simulink model "BEVplantModel"  (R2022b)
settings: Solver=daessc  StartTime=0  StopTime=50  RelTol=1e-3
PreLoadFcn:
  | % Load all parameters
  | BEVplantModelParam;
undefined symbols (not defined in the file): battery, cabin_T_init, coolant_pipe_D, coolant_valve_D_ratio_max, coolant_valve_D_ratio_min, coolant_valve_displacement, electricDrive, max_torque, vehicle, vehicleThermal
libraries: fl_lib x292, nesl_utility x67, SimscapeFluids_lib x15, ee_lib x11, sdl_lib x8, BatteryCurrentManagement x3, slpidlib x3, simulink x2, BatteryThermalManagement x1, autolibshared x1
(part 5 of 10)

== system BEVplantModel/Vehicle/Rear Motor (EM2) ==
  s : Inport
  Bus Creator : BusCreator  Inputs=2
  Bus Selector : BusSelector  OutputSignals=EM2Trq,Batt
  Bus Selector1 : BusSelector  OutputSignals=EM1rpm
  Coolant Jacket : SimscapeFluids_lib/Thermal Liquid/Pipes & Fittings/Pipe (TL)  dynamic_compressibility=1  inertia=0  num_segments=1  pipe_length=0.4 m  area=4 * pi * vehicleThermal.coolant_channel_D^2 / 4 m^2  wall_spec=1  Dh=vehicleThermal.coolant_channel_D m  wall_compliance=1.2e-6 m/MPa  wall_time_constant=0.01 s  elevation_spec=foundation.enum.constant_variable.constant  elevation_gain=0 m  g=9.81 m/s^2  pressure_loss_spec=1  local_pressure_loss_spec=fluids.thermal_liquid.pipes_fittings.enum.LocalLossSpec.AggregateLength  length_add=20 * vehicleThermal.coolant_channel_D * 4 m  loss_coefficient=0.1  roughness=1.5e-5 m  Re_friction_TLU=[ 400 1000 1.5e+3 3e+3 4e+3 6e+3 1e+4 2e+4 4e+4 6e+4 1e+5 1e+8 ]  friction_factor_TLU=[ 0.264 0.112 0.07099999999999999 0.0417 0.0387 0.0268 0.025 0.0232 0.0226 0.022 0.0214 0.0214 ]  shape_factor=64  Re_lam=100  Re_tur=500  mdot_nominal=[ 0.1 1 ] kg/s  p_diff_nominal=[ 0.001 0.01 ] MPa  mdot_threshold=1e-6 kg/s  heat_transfer_spec=4  mdot_nominal_heat=[ 0.1 1 ] kg/s  T_in_nominal=[ 293.15 293.15 ] K  T_out_nominal=[ 300 300 ] K  p_in_nominal_heat=[ 0.101325 0.101325 ] MPa  T_wall_nominal=[ 303.15 303.15 ] K  a_coeff=0.3  b_Re_power=0.8  c_Pr_power=0.33  Nu_lam=3.66  Re_Colburn_TLU=[ 100 150 1000 ]  Colburn_factor_TLU=[ 0.019 0.013 0.002 ]  Re_Nu_TLU=[ 100 150 1000 ]  Pr_Nu_TLU=[ 1 10 ]  Nu_TLU=[ 3.72 4.21; 3.75 4.44; 4.21 7.15 ]  T0_vec=vehicleThermal.coolant_T_init K  p0_vec=vehicleThermal.coolant_p_init MPa  mdot0=0.1 kg/s
  Emotor : Subsystem
      settings: PortSchema="{\"entries\":[{\"content\":{\"sides\":[{\"content\":{\"connectorIds\":[\"LConn1\",\"In1\"]},\"type\":\"ConnectorPlacement.EquallySpacedRectSide\",\"uuid\":\"4c01f4e7-db0d-4a8e-9bf8-0007797f2983\"},{\"content\":{\"connectorIds\":[\"RConn1\",\"Out1\",\"RConn2\"],\"side\":\"RIGHT\"},\"type\":\"ConnectorPlacement.EquallySpacedRectSide\",\"uuid\":\"016ff73d-d921-4c23-b0f0-ceb092773eb0\"},{\"content\":{\"connectorIds\":[],\"side\":\"TOP\"},\"type\":\"ConnectorPlacement.EquallySpacedRectSide\",\"uuid\":\"4629c7d5-cdf8-4573-9adc-69c84e237e94\"}]},\"type\":\"ConnectorPlacement.EquallySpacedConnector\",\"uuid\":\"4efbbf6b-ce98-44e7-ad85-9bcf934dac12\"}],\"packageUris\":[\"http://schema.mathworks.com/mf0/Connector/R2020b\"],\"version\":\"1.0\"}"
  Emotor Input : Subsystem
  Emotor Output : Subsystem
  Inverter Pipe : SimscapeFluids_lib/Thermal Liquid/Pipes & Fittings/Pipe (TL)  dynamic_compressibility=1  inertia=0  num_segments=1  pipe_length=0.4 m  area=4 * pi * vehicleThermal.coolant_channel_D^2 / 4 m^2  wall_spec=1  Dh=vehicleThermal.coolant_channel_D m  wall_compliance=1.2e-6 m/MPa  wall_time_constant=0.01 s  elevation_spec=foundation.enum.constant_variable.constant  elevation_gain=0 m  g=9.81 m/s^2  pressure_loss_spec=1  local_pressure_loss_spec=fluids.thermal_liquid.pipes_fittings.enum.LocalLossSpec.AggregateLength  length_add=20 * vehicleThermal.coolant_channel_D * 4 m  loss_coefficient=0.1  roughness=1.5e-5 m  Re_friction_TLU=[ 400 1000 1.5e+3 3e+3 4e+3 6e+3 1e+4 2e+4 4e+4 6e+4 1e+5 1e+8 ]  friction_factor_TLU=[ 0.264 0.112 0.07099999999999999 0.0417 0.0387 0.0268 0.025 0.0232 0.0226 0.022 0.0214 0.0214 ]  shape_factor=64  Re_lam=100  Re_tur=500  mdot_nominal=[ 0.1 1 ] kg/s  p_diff_nominal=[ 0.001 0.01 ] MPa  mdot_threshold=1e-6 kg/s  heat_transfer_spec=4  mdot_nominal_heat=[ 0.1 1 ] kg/s  T_in_nominal=[ 293.15 293.15 ] K  T_out_nominal=[ 300 300 ] K  p_in_nominal_heat=[ 0.101325 0.101325 ] MPa  T_wall_nominal=[ 303.15 303.15 ] K  a_coeff=0.3  b_Re_power=0.8  c_Pr_power=0.33  Nu_lam=3.66  Re_Colburn_TLU=[ 100 150 1000 ]  Colburn_factor_TLU=[ 0.019 0.013 0.002 ]  Re_Nu_TLU=[ 100 150 1000 ]  Pr_Nu_TLU=[ 1 10 ]  Nu_TLU=[ 3.72 4.21; 3.75 4.44; 4.21 7.15 ]  T0_vec=vehicleThermal.coolant_T_init K  p0_vec=vehicleThermal.coolant_p_init MPa  mdot0=0.1 kg/s
  Inverter Power Module Thermal : Subsystem
  SC1 : Subsystem
      mask Display: disp(get_param(gcb, 'Name'))
  Simulink-PS Converter : nesl_utility/Simulink-PS Converter  PhysicalDomain=network_engine_domain  SubClassName=ps_input  LeftPortType=input  RightPortType=output  PseudoPeriodic=off  Frequencies=[]  NoiseDistribution=none  NoiseParameters=[]  Unit=rpm  AffineConversion=off  FilteringAndDerivatives=provide  SimscapeFilterOrder=1  InputFilterTimeConstant=0.001  UdotUserProvided=0
  Simulink-PS Converter1 : nesl_utility/Simulink-PS Converter  PhysicalDomain=network_engine_domain  SubClassName=ps_input  LeftPortType=input  RightPortType=output  PseudoPeriodic=off  Frequencies=[]  NoiseDistribution=none  NoiseParameters=[]  Unit=N*m  AffineConversion=off  FilteringAndDerivatives=provide  SimscapeFilterOrder=1  InputFilterTimeConstant=0.001  UdotUserProvided=0
  Transfer Fcn3 : TransferFcn  Denominator=[0.01 1]
  m3/s to m/s : Subsystem
  HV : PMIOPort  Side=Left
  A : PMIOPort  Port=2  Side=Left
  Ax : PMIOPort  Port=3  Side=Right
  B : PMIOPort  Port=4  Side=Right
  m : Outport
  wires:
  Bus Selector/1 -> [Tq], Emotor Input/1(TrqCmd)  "<EM2Trq>"
  Bus Selector/2 -> Emotor Input/2(" Batt")  "<Batt>"
  Emotor/1(S) -> Emotor Output/1(S), [sens]
  Emotor Input/1(EMctl) -> Emotor/1(EMctl)
  Bus Creator/1 -> m/1
  Emotor Output/1(EM2) -> Bus Creator/1  "EM2"
  Emotor Output/2(E) -> Bus Creator/2  "EM2energy"
  s/1 -> Bus Selector/1
  [Tq] -> Simulink-PS Converter1/1
  [sens] -> Bus Selector1/1
  Bus Selector1/1 -> Transfer Fcn3/1  "<EM1rpm>"
  Transfer Fcn3/1 -> Simulink-PS Converter/1
  connections:
  Emotor/RConn1 -- Ax/RConn1
  Emotor/LConn1 -- HV/RConn1
  Inverter Pipe/LConn1 -- Coolant Jacket/RConn1
  m3/s to m/s/RConn1 -- Inverter Power Module Thermal/LConn1
  Simulink-PS Converter1/RConn1 -- Inverter Power Module Thermal/LConn3
  SC1/LConn1 -- B/RConn1
  Inverter Power Module Thermal/RConn1 -- Inverter Pipe/LConn2
  Coolant Jacket/LConn1 -- SC1/RConn1
  A/RConn1 -- Inverter Pipe/RConn1
  Coolant Jacket/LConn2 -- Emotor/RConn2
  m3/s to m/s/LConn1 -- SC1/RConn2
  Simulink-PS Converter/RConn1 -- Inverter Power Module Thermal/LConn2

== system BEVplantModel/Controller/BMS/Battery Protection Logic ==
  Current : Inport
  Sensor : Inport  Port=2
  SoC : Inport  Port=3
  State Flow : Subsystem  mask{MinVoltLmt=battery.MinVoltLmt, MaxVoltLmt=battery.MaxVoltLmt, VoltOffset=battery.VoltOffset, CurrOffset=battery.CurrOffset, MinThLmt=battery.MinThLmt, MaxThLmt=battery.MaxThLmt}
      mask prompts: MinVoltLmt "Minimum Voltage Limit"; MaxVoltLmt "Maximum Voltage Limit"; VoltOffset "Voltage fault offset"; CurrOffset "Current fault offset"; MinThLmt "Min cell temp"; MaxThLmt "Max cell temp"
      mask DialogControl ParameterGroupVar Prompt: Battery Fault Parameters
  Stateflow Input : Subsystem
  StateOut : Outport
  wires:
  State Flow/1(StateOut) -> StateOut/1
  Stateflow Input/1(StateInput) -> State Flow/1(StateInput)
  SoC/1 -> Stateflow Input/1(SoC)
  Current/1 -> Stateflow Input/2(Current)
  Sensor/1 -> Stateflow Input/3(Sensor)

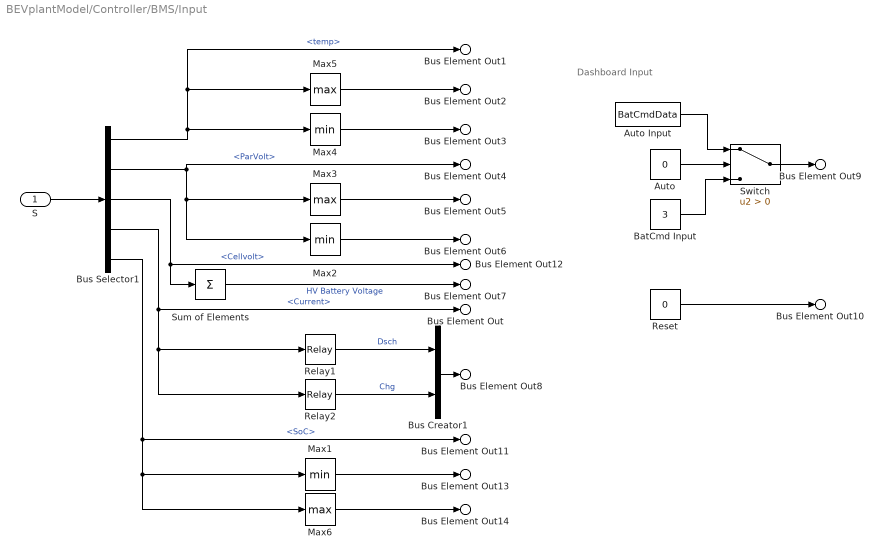
== system BEVplantModel/Controller/BMS/Input ==
  note: Dashboard Input
  S : Inport
  Auto : Constant  Value=0
  Auto Input : FromWorkspace  VariableName=BatCmdData
  BatCmd Input : Constant  Value=3
  Bus Creator1 : BusCreator  Inputs=2
  Bus Selector1 : BusSelector  OutputSignals=temp,ParVolt,Cellvolt,Current,SoC
  Max1 : MinMax  ZeroCross=off
  Max2 : MinMax  ZeroCross=off
  Max3 : MinMax  Function=max  ZeroCross=off
  Max4 : MinMax  ZeroCross=off
  Max5 : MinMax  Function=max  ZeroCross=off
  Max6 : MinMax  Function=max  ZeroCross=off
  Relay1 : Relay  OnSwitchValue=0  OffSwitchValue=-5  OnOutputValue=0  OffOutputValue=1  ZeroCross=off
  Relay2 : Relay  OnSwitchValue=5  OffSwitchValue=0  ZeroCross=off
  Reset : Constant  Value=0
  Sum of Elements : Sum  Inputs=+
  Switch : Switch  Criteria=u2 > Threshold  SaturateOnIntegerOverflow=off  InputSameDT=off
  Bus Element Out : Outport  PortName=BatData  Element=Cur
  Bus Element Out1 : Outport  PortName=BatData  Element=CellTemp
  Bus Element Out2 : Outport  PortName=BatData  Element=CellTempMax
  Bus Element Out3 : Outport  PortName=BatData  Element=CellTempMin
  Bus Element Out4 : Outport  PortName=BatData  Element=CellVolt
  Bus Element Out5 : Outport  PortName=BatData  Element=CellVoltMax
  Bus Element Out6 : Outport  PortName=BatData  Element=CellVoltMin
  Bus Element Out7 : Outport  PortName=BatData  Element=BatVolt
  Bus Element Out8 : Outport  PortName=BatData  Element=CurDir
  Bus Element Out11 : Outport  PortName=BatData  Element=SoC
  Bus Element Out12 : Outport  PortName=BatData  Element=BatParVolt
  Bus Element Out13 : Outport  PortName=BatData  Element=minSoC
  Bus Element Out14 : Outport  PortName=BatData  Element=maxSoC
  Bus Element Out9 : Outport  PortName=BatData  Element=BatCmd
  Bus Element Out10 : Outport  PortName=BatData  Element=Reset
  wires:
  Bus Selector1/5 -> Bus Element Out11/1, Max1/1, Max6/1  "<SoC>"
  Bus Selector1/3 -> Sum of Elements/1, Bus Element Out12/1  "<Cellvolt>"
  Relay1/1 -> Bus Creator1/1  "Dsch"
  Bus Selector1/1 -> Bus Element Out1/1, Max5/1, Max4/1  "<temp>"
  Bus Selector1/4 -> Bus Element Out/1, Relay1/1, Relay2/1  "<Current>"
  Sum of Elements/1 -> Bus Element Out7/1  "HV Battery Voltage"
  S/1 -> Bus Selector1/1
  Bus Selector1/2 -> Bus Element Out4/1, Max3/1, Max2/1  "<ParVolt>"
  Auto/1 -> Switch/2
  Auto Input/1 -> Switch/1
  Reset/1 -> Bus Element Out10/1
  BatCmd Input/1 -> Switch/3
  Switch/1 -> Bus Element Out9/1
  Max5/1 -> Bus Element Out2/1
  Max4/1 -> Bus Element Out3/1
  Max3/1 -> Bus Element Out5/1
  Max2/1 -> Bus Element Out6/1
  Bus Creator1/1 -> Bus Element Out8/1
  Relay2/1 -> Bus Creator1/2  "Chg"
  Max1/1 -> Bus Element Out13/1
  Max6/1 -> Bus Element Out14/1

== system BEVplantModel/Controller/BMS/MinMax Current Limiter ==
  Bus Element In3 : Inport  PortName=Sensor  Element=Cur
  Bus Element In1 : Inport  PortName=Sensor  Element=Cur
  Bus Element In10 : Inport  PortName=Sensor  Element=Cur
  Bus Element In2 : Inport  PortName=Sensor  Element=CellVoltMin
  Bus Element In8 : Inport  PortName=Sensor  Element=CellVoltMax
  Bus Element In9 : Inport  PortName=Sensor  Element=CurDir
  Bus Element In5 : Inport  PortName=Sensor  Element=CellTempMin
  Bus Element In7 : Inport  PortName=Sensor  Element=CellTempMin
  Bus Element In4 : Inport  PortName=Sensor  Element=CellTempMax
  Bus Element In6 : Inport  PortName=Sensor  Element=CellTempMax
  Current Directional : Subsystem
  OCprotection : Subsystem
  ODprotection : Subsystem
  Bus Element Out : Outport  PortName=Current  Element=CurDchLmt
  Bus Element Out1 : Outport  PortName=Current  Element=CurChgLmt
  Bus Element Out2 : Outport  PortName=Current  Element=CurDchWarn
  Bus Element Out3 : Outport  PortName=Current  Element=CurChgWarn
  Bus Element Out4 : Outport  PortName=Current  Element=CurChgDchg
  wires:
  ODprotection/2(ODWarn) -> Bus Element Out2/1
  Bus Element In8/1 -> OCprotection/2(VoltMax)
  Bus Element In2/1 -> ODprotection/2(VoltMin)
  OCprotection/1(OCWarn) -> Bus Element Out3/1
  Bus Element In6/1 -> OCprotection/3(CellTpMax)
  Bus Element In7/1 -> OCprotection/4(CellTpMin)
  Bus Element In9/1 -> Current Directional/1(CurDir)
  Bus Element In4/1 -> ODprotection/3(CellTpMax)
  Bus Element In5/1 -> ODprotection/4(CellTpMin)
  ODprotection/1(DschCurLim) -> Bus Element Out/1
  OCprotection/2(ChrgCurLim) -> Bus Element Out1/1
  Bus Element In3/1 -> ODprotection/1(Cur)
  Bus Element In1/1 -> OCprotection/1(Cur)
  Current Directional/1(I_Current) -> Bus Element Out4/1
  Bus Element In10/1 -> Current Directional/2(Cur)

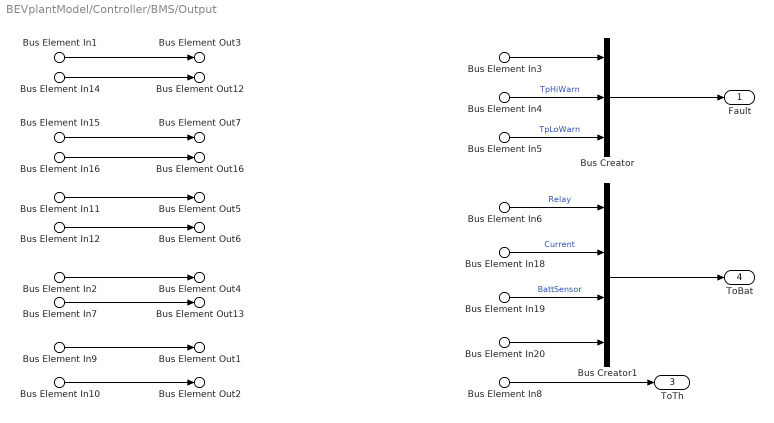
== system BEVplantModel/Controller/BMS/Output ==
  Bus Element In19 : Inport  PortName=BatData
  Bus Element In9 : Inport  PortName=BatData  Element=Cur
  Bus Element In10 : Inport  PortName=BatData  Element=BatVolt
  Bus Element In11 : Inport  PortName=BatData  Element=CellTempMax
  Bus Element In12 : Inport  PortName=BatData  Element=CellTempMin
  Bus Element In18 : Inport  Port=2  PortName=Current
  Bus Element In2 : Inport  Port=2  PortName=Current  Element=CurChgLmt
  Bus Element In7 : Inport  Port=2  PortName=Current  Element=CurDchLmt
  Bus Element In3 : Inport  Port=3  PortName=StateOut  Element=Fault
  Bus Element In6 : Inport  Port=3  PortName=StateOut  Element=RelayRq
  Bus Element In20 : Inport  Port=3  PortName=StateOut  Element=BatSt
  Bus Element In1 : Inport  Port=4  PortName=SoC  Element=CellSoCmax
  Bus Element In14 : Inport  Port=4  PortName=SoC  Element=CellSoCmin
  Bus Element In8 : Inport  Port=5  PortName=Thermal
  Bus Element In{4..5,15..16} (4 alike) : Inport  Port=5  PortName=Thermal  Element=TpHiWarning
  Bus Creator : BusCreator  Inputs=3
  Bus Creator1 : BusCreator  Inputs=4
  Fault : Outport
  Bus Element Out3 : Outport  Port=2  PortName=plot  Element=SoCMax
  Bus Element Out4 : Outport  Port=2  PortName=plot  Element=CurChgLmt
  Bus Element Out7 : Outport  Port=2  PortName=plot  Element=HiThWarn
  Bus Element Out12 : Outport  Port=2  PortName=plot  Element=SoCMin
  Bus Element Out13 : Outport  Port=2  PortName=plot  Element=CurDchgLmt
  Bus Element Out16 : Outport  Port=2  PortName=plot  Element=LoThWarn
  Bus Element Out1 : Outport  Port=2  PortName=plot  Element=Cur
  Bus Element Out2 : Outport  Port=2  PortName=plot  Element=BatVolt
  Bus Element Out5 : Outport  Port=2  PortName=plot  Element=TpMax
  Bus Element Out6 : Outport  Port=2  PortName=plot  Element=TpMin
  ToTh : Outport  Port=3
  ToBat : Outport  Port=4
  wires:
  Bus Creator/1 -> Fault/1
  Bus Creator1/1 -> ToBat/1
  Bus Element In18/1 -> Bus Creator1/2  "Current"
  Bus Element In12/1 -> Bus Element Out6/1
  Bus Element In11/1 -> Bus Element Out5/1
  Bus Element In10/1 -> Bus Element Out2/1
  Bus Element In8/1 -> ToTh/1
  Bus Element In9/1 -> Bus Element Out1/1
  Bus Element In6/1 -> Bus Creator1/1  "Relay"
  Bus Element In5/1 -> Bus Creator/3  "TpLoWarn"
  Bus Element In4/1 -> Bus Creator/2  "TpHiWarn"
  Bus Element In3/1 -> Bus Creator/1
  Bus Element In14/1 -> Bus Element Out12/1
  Bus Element In2/1 -> Bus Element Out4/1
  Bus Element In1/1 -> Bus Element Out3/1
  Bus Element In7/1 -> Bus Element Out13/1
  Bus Element In15/1 -> Bus Element Out7/1
  Bus Element In16/1 -> Bus Element Out16/1
  Bus Element In19/1 -> Bus Creator1/3  "BattSensor"
  Bus Element In20/1 -> Bus Creator1/4

== system BEVplantModel/Controller/BMS/Thermal Management ==
  Bus Element In3 : Inport  PortName=Sensor  Element=CellTempMin
  Bus Element In1 : Inport  PortName=Sensor  Element=CellTempMax
  Bus Element In4 : Inport  PortName=Sensor  Element=CellTemp
  Ambient : Constant  Value=vehicleThermal.ambient
  Battery Coolant Control : BatteryThermalManagement/Battery Coolant Control  ControlStrategy=ON-OFF control  TempOn=battery.CoolantSwitchOnTp  TempOff=battery.CoolantSwitchOffTp  c=0.1  FlowRateStep=0.2
      settings: LibrarySourceBlock=batt_sl_lib/Thermal Management/Battery Coolant Control
  CoolantTp : Constant  Value=vehicleThermal.coolant_T_init
  Terminator : Terminator
  Transfer Fcn : TransferFcn  Denominator=[1 1]
  Warning <283K : Relay  OnSwitchValue=290  OffSwitchValue=283  OnOutputValue=0  OffOutputValue=1
  Warning >300K : Relay  OnSwitchValue=320  OffSwitchValue=310
  Bus Element Out1 : Outport  PortName=Thermal  Element=CoolFlow
  Bus Element Out3 : Outport  PortName=Thermal  Element=TpHiWarning
  Bus Element Out4 : Outport  PortName=Thermal  Element=TpLoWarning
  wires:
  Battery Coolant Control/2 -> Terminator/1
  Bus Element In4/1 -> Battery Coolant Control/3
  Transfer Fcn/1 -> Bus Element Out1/1
  CoolantTp/1 -> Battery Coolant Control/2  "Min"
  Ambient/1 -> Battery Coolant Control/1  "Min"
  Bus Element In3/1 -> Warning <283K/1
  Bus Element In1/1 -> Warning >300K/1
  Warning <283K/1 -> Bus Element Out4/1  "TpLowWarn"
  Warning >300K/1 -> Bus Element Out3/1  "TpHighWarn"
  Battery Coolant Control/1 -> Transfer Fcn/1

== system BEVplantModel/Controller/Output/Battery ==
  Batt : Inport
  BA : Outport
  wires:
  Batt/1 -> BA/1  "BA"

== system BEVplantModel/Controller/Output/BatteryPump ==
  ThCtrl : Inport
  Batt : Inport  Port=2
  Bus Creator : BusCreator  Inputs=2
  Bus Selector : BusSelector  OutputSignals=BatSt
  Bus Selector1 : BusSelector  OutputSignals=cmdBatteryPump
  BP : Outport
  wires:
  Bus Selector1/1 -> Bus Creator/1  "<cmdBatteryPump>"
  ThCtrl/1 -> Bus Selector1/1
  Bus Creator/1 -> BP/1  "BP"
  Batt/1 -> Bus Selector/1
  Bus Selector/1 -> Bus Creator/2  "<BatSt>"

== system BEVplantModel/Controller/Output/Charger ==
  Batt : Inport
  Bus Creator : BusCreator  Inputs=1
  CG : Outport
  wires:
  Batt/1 -> Bus Creator/1  "Batt"
  Bus Creator/1 -> CG/1  "CG"

== system BEVplantModel/Controller/Output/Chiller ==
  Batt : Inport
  ThCtrl : Inport  Port=2
  Bus Creator2 : BusCreator  Inputs=2
  Bus Selector4 : BusSelector  OutputSignals=cmdChillerByp
  CH : Outport
  wires:
  Bus Selector4/1 -> Bus Creator2/2  "<cmdChillerByp>"
  Bus Creator2/1 -> CH/1  "CH"
  Batt/1 -> Bus Creator2/1
  ThCtrl/1 -> Bus Selector4/1

== system BEVplantModel/Controller/Output/ChillerValve ==
  ThCtrl : Inport
  Bus Selector3 : BusSelector  OutputSignals=cmdChillerByp
  Gain3 : Gain
  CV : Outport
  wires:
  Bus Selector3/1 -> Gain3/1  "<cmdChillerByp>"
  ThCtrl/1 -> Bus Selector3/1
  Gain3/1 -> CV/1  "CV"

== system BEVplantModel/Controller/Output/ControlValve ==
  Env : Inport
  ThCtrl : Inport  Port=2
  Bus Creator : BusCreator  Inputs=2
  Bus Selector : BusSelector  OutputSignals=Tenv
  Bus Selector1 : BusSelector  OutputSignals=cmdParallelSerieal
  MV : Outport
  wires:
  Env/1 -> Bus Selector/1
  Bus Selector/1 -> Bus Creator/1  "<Tenv>"
  Bus Selector1/1 -> Bus Creator/2  "<cmdParallelSerieal>"
  Bus Creator/1 -> MV/1  "MV"
  ThCtrl/1 -> Bus Selector1/1

== system BEVplantModel/Controller/Output/EM1 ==
  TrqCmd : Inport
  Batt : Inport  Port=2
  Bus Creator3 : BusCreator  Inputs=2
  Bus Selector1 : BusSelector  OutputSignals=EM1Trq
  M1 : Outport
  wires:
  Bus Selector1/1 -> Bus Creator3/1  "<EM1Trq>"
  Bus Creator3/1 -> M1/1  "M1"
  Batt/1 -> Bus Creator3/2
  TrqCmd/1 -> Bus Selector1/1

== system BEVplantModel/Controller/Output/EM2 ==
  Batt : Inport
  TrqCmd : Inport  Port=2
  Bus Creator2 : BusCreator  Inputs=2
  Bus Selector : BusSelector  OutputSignals=EM2Trq
  M2 : Outport
  wires:
  TrqCmd/1 -> Bus Selector/1
  Bus Selector/1 -> Bus Creator2/1  "<EM2Trq>"
  Bus Creator2/1 -> M2/1  "M2"
  Batt/1 -> Bus Creator2/2

== system BEVplantModel/Controller/Output/HVAC ==
  Env : Inport
  Batt : Inport  Port=2
  Cabin : Inport  Port=3
  Bus Creator : BusCreator  Inputs=4
  Bus Selector4 : BusSelector  OutputSignals=Tenv
  Bus Selector5 : BusSelector  OutputSignals=TpSetPoint,acOnOff
  VA : Outport
  wires:
  Bus Selector5/2 -> Bus Creator/4  "<acOnOff>"
  Bus Creator/1 -> VA/1  "VA"
  Cabin/1 -> Bus Selector5/1
  Bus Selector4/1 -> Bus Creator/1  "<Tenv>"
  Bus Selector5/1 -> Bus Creator/3  "<TpSetPoint>"
  Batt/1 -> Bus Creator/2
  Env/1 -> Bus Selector4/1

== system BEVplantModel/Controller/Output/Heater ==
  ThCtrl : Inport
  Batt : Inport  Port=2
  Bus Creator : BusCreator  Inputs=2
  Bus Selector3 : BusSelector  OutputSignals=cmdHeater
  HE : Outport
  wires:
  ThCtrl/1 -> Bus Selector3/1
  Bus Selector3/1 -> Bus Creator/2  "<cmdHeater>"
  Bus Creator/1 -> HE/1  "HE"
  Batt/1 -> Bus Creator/1

== system BEVplantModel/Controller/Output/MotorPump ==
  ThCtrl : Inport
  Batt : Inport  Port=2
  Bus Creator : BusCreator  Inputs=2
  Bus Selector : BusSelector  OutputSignals=cmdMotorPump
  Bus Selector1 : BusSelector  OutputSignals=BatSt
  MP : Outport
  wires:
  Bus Selector/1 -> Bus Creator/1  "<cmdMotorPump>"
  ThCtrl/1 -> Bus Selector/1
  Bus Creator/1 -> MP/1  "MP"
  Batt/1 -> Bus Selector1/1
  Bus Selector1/1 -> Bus Creator/2  "<BatSt>"

== system BEVplantModel/Controller/Output/Radiator ==
  Env : Inport
  VehSpd : Inport  Port=2
  ThCtrl : Inport  Port=3
  Bus Creator : BusCreator  Inputs=3
  Bus Selector : BusSelector  OutputSignals=cmdFan
  RA : Outport
  wires:
  Bus Selector/1 -> Bus Creator/3  "<cmdFan>"
  Bus Creator/1 -> RA/1  "RA"
  ThCtrl/1 -> Bus Selector/1
  VehSpd/1 -> Bus Creator/2
  Env/1 -> Bus Creator/1  "Env"

== system BEVplantModel/Controller/Output/RadiatorByp ==
  ThCtrl : Inport
  Bus Selector2 : BusSelector  OutputSignals=cmdRadByp
  Gain : Gain
  RV : Outport
  wires:
  Bus Selector2/1 -> Gain/1  "<cmdRadByp>"
  ThCtrl/1 -> Bus Selector2/1
  Gain/1 -> RV/1  "RV"

== system BEVplantModel/Controller/Range Estimator/Distance ==
  VehSpd : Inport
  Add : Sum
  Constant : Constant
  Constant1 : Constant  Value=0.1
  Display : Display
  Divide : Product  Inputs=*/
  Gain : Gain  Gain=1/3.6
  Gain1 : Gain  Gain=1/1000
  Gain2 : Gain  Gain=3.6
  Integrator : Integrator
  Integrator1 : Integrator
  Dist : Outport
  SimTime(s) : Outport  Port=2
  wires:
  Constant/1 -> Integrator1/1
  VehSpd/1 -> Gain/1
  Integrator/1 -> Gain1/1, Divide/1
  Constant1/1 -> Add/2
  Integrator1/1 -> Add/1  "time"
  Add/1 -> Divide/2, SimTime(s)/1
  Divide/1 -> Gain2/1
  Gain/1 -> Integrator/1
  Gain1/1 -> Dist/1  "Distance"
  Gain2/1 -> Display/1

== system BEVplantModel/Controller/Range Estimator/Online Range ==
  d : Inport
  s : Inport  Port=2
  Bus Selector : BusSelector  OutputSignals=Batt.BattSensor.minSoC,Batt.BattSensor.BatVolt,Batt.BattSensor.Cur
  Constant1 : Constant  Value=battery.AH*400*battery.Np
  Constant5 : Constant  Value=500
  Divide1 : Product  Inputs=*/
  Energy Consumption : Subsystem
  Max1 : MinMax  Inputs=2
  Product1 : Product
  Subsystem : Subsystem
  E : Outport
  RangeOnline : Outport  Port=2
  wires:
  Bus Selector/1 -> Product1/2  "<minSoC>"
  Constant5/1 -> Max1/2
  Divide1/1 -> Max1/1
  Max1/1 -> RangeOnline/1
  s/1 -> Bus Selector/1
  Energy Consumption/1(E) -> Subsystem/1(E), E/1  "Energy"
  Bus Selector/2 -> Energy Consumption/1(V)  "<BatVolt>"
  Bus Selector/3 -> Energy Consumption/2(I)  "<Cur>"
  Constant1/1 -> Product1/1
  Product1/1 -> Divide1/1
  d/1 -> Subsystem/2(d)
  Subsystem/1(E/D) -> Divide1/2  "E/D"

== system BEVplantModel/Controller/Range Estimator/Range Rating ==
  note: Total capacity at full charge , Ahr*BatVoltage*CellinSeries
  d : Inport
  E : Inport  Port=2
  Add : Sum
  Constant : Constant
  Display : Display
  Divide : Product  Inputs=*/
  Divide1 : Product  Inputs=/*
  TotalEnergy : Constant  Value=battery.AH*400*battery.Np
  wires:
  Add/1 -> Divide1/1
  Constant/1 -> Add/1
  E/1 -> Divide/1
  d/1 -> Divide/2
  Divide1/1 -> Display/1  "RangeRating"
  Divide/1 -> Add/2
  TotalEnergy/1 -> Divide1/2

== system BEVplantModel/Controller/Thermal Control/Coolant Control ==
  T_env : Inport
  T_coolant_battery_in : Inport  Port=2
  T_motor : Inport  Port=3
  T_battery : Inport  Port=4
  T_coolant_motor_out : Inport  Port=5
  Battery Heater : Subsystem
  Battery Pump : Subsystem
  Chiller Bypass : Subsystem
  Motor Pump : Subsystem
  Parallel-Serial Mode : Subsystem
  Radiator Bypass : Subsystem
  cmd_heater : Outport
  cmd_motor_pump : Outport  Port=2
  cmd_battery_pump : Outport  Port=3
  cmd_chiller_bypass : Outport  Port=4
  cmd_parallel_serial : Outport  Port=5
  cmd_rad_bypass : Outport  Port=6
  wires:
  T_battery/1 -> Battery Pump/2(T_battery), Chiller Bypass/1(T_battery)
  Chiller Bypass/1(cmd_chiller_bypass) -> cmd_chiller_bypass/1, Parallel-Serial Mode/1(cmd_chiller_bypass), Battery Pump/3(cmd_chiller_bypass)
  Radiator Bypass/1(cmd_rad_bypass) -> cmd_rad_bypass/1
  Battery Pump/1(cmd_battery_pump) -> cmd_battery_pump/1
  Battery Heater/1(cmd_heater) -> cmd_heater/1
  T_motor/1 -> Motor Pump/1(T_motor)
  T_coolant_motor_out/1 -> Radiator Bypass/1(T_coolant_motor_out), Parallel-Serial Mode/3(T_coolant_motor_out)
  T_coolant_battery_in/1 -> Battery Heater/2(T_coolant_battery_in)
  T_env/1 -> Parallel-Serial Mode/2(T_env), Battery Heater/1(T_env)
  Motor Pump/1(cmd_motor_pump) -> cmd_motor_pump/1, Battery Pump/1(cmd_motor_pump)
  Parallel-Serial Mode/1(cmd_parallel_serial) -> Battery Pump/4(parallel_serial), cmd_parallel_serial/1

== system BEVplantModel/Controller/Thermal Control/Fan Control ==
  T_motor : Inport
  Motor Requirement : Subsystem
  cmd_fan : Outport
  wires:
  T_motor/1 -> Motor Requirement/1(T_motor)
  Motor Requirement/1(cmd_fan) -> cmd_fan/1

== system BEVplantModel/Controller/Vehicle Control/Driver ==
  VehSpdRef : Inport
  rpm : Inport  Port=2
  Motor Speed Reference : Subsystem
  Speed Controller : Subsystem
      settings: PortSchema="{\"entries\":[{\"content\":{\"sides\":[{\"content\":{\"connectorIds\":[\"Out1\"]},\"type\":\"ConnectorPlacement.EquallySpacedRectSide\",\"uuid\":\"12b9f2c9-2b28-451b-ad36-7fe4150db485\"},{\"content\":{\"connectorIds\":[\"In2\"],\"side\":\"RIGHT\"},\"type\":\"ConnectorPlacement.EquallySpacedRectSide\",\"uuid\":\"c0fdf9a4-483a-4ddc-b663-6299fcc79327\"},{\"content\":{\"connectorIds\":[\"In1\"],\"side\":\"TOP\"},\"type\":\"ConnectorPlacement.EquallySpacedRectSide\",\"uuid\":\"3f20082e-8487-45e3-9fd7-d6d75741df4d\"}]},\"type\":\"ConnectorPlacement.EquallySpacedConnector\",\"uuid\":\"9361cdd3-74d8-46ee-ae7f-e2dde5d31ed1\"}],\"packageUris\":[\"http://schema.mathworks.com/mf0/Connector/19700101\"],\"version\":\"1.0\"}"
  TrqReq : Outport
  wires:
  Motor Speed Reference/1(MotorSpdRef) -> Speed Controller/2(SpdRef)
  rpm/1 -> Speed Controller/1(Spd)
  Speed Controller/1(TrqPID) -> TrqReq/1
  VehSpdRef/1 -> Motor Speed Reference/1(VehSpd)

== system BEVplantModel/Controller/Vehicle Control/Torque Control ==
  TrqReq : Inport
  Crtl : Inport  Port=2
  Brake/Motor Trq Split : Subsystem
      settings: PortSchema="{\"entries\":[{\"content\":{\"sides\":[{\"content\":{\"connectorIds\":[\"In1\",\"In2\",\"In3\"]},\"type\":\"ConnectorPlacement.EquallySpacedRectSide\",\"uuid\":\"c6883188-188e-4cbf-9dc5-1a26bf01b714\"},{\"content\":{\"connectorIds\":[\"Out1\"],\"side\":\"RIGHT\"},\"type\":\"ConnectorPlacement.EquallySpacedRectSide\",\"uuid\":\"b7c90991-838b-485d-9a4c-3fbacac28b54\"},{\"content\":{\"connectorIds\":[\"Out2\"],\"side\":\"TOP\"},\"type\":\"ConnectorPlacement.EquallySpacedRectSide\",\"uuid\":\"50e43671-3241-4bf5-a3b9-e23b27b7214a\"},{\"content\":{\"connectorIds\":[],\"side\":\"HIDDEN\"},\"type\":\"ConnectorPlacement.EquallySpacedRectSide\",\"uuid\":\"7c25a71e-e9cc-425c-8a3d-1b4aa412427f\"}]},\"type\":\"ConnectorPlacement.EquallySpacedConnector\",\"uuid\":\"d51dcaef-c892-4ef2-982d-c6c52760ceaa\"}],\"packageUris\":[\"http://schema.mathworks.com/mf0/Connector/R2020b\"],\"version\":\"1.0\"}"
  Bus Creator1 : BusCreator  Inputs=2
  Bus Creator3 : BusCreator  Inputs=4
  Bus Creator4 : BusCreator  Inputs=2
  Bus Selector : BusSelector  OutputSignals=m.M1.EM1.EM1rpm,Batt.BattSensor.BatVolt,Batt.BattSensor.CellTemp,Batt.BattSensor.maxSoC
  Charge/Discharge Limit : Subsystem
  Mech. Brake Model : Subsystem
      settings: PortSchema="{\"entries\":[{\"content\":{\"sides\":[{\"content\":{\"connectorIds\":[\"In1\"]},\"type\":\"ConnectorPlacement.EquallySpacedRectSide\",\"uuid\":\"3fcf8e06-a346-49b8-a4a8-b41cf2b27013\"},{\"content\":{\"connectorIds\":[\"Out1\"],\"side\":\"RIGHT\"},\"type\":\"ConnectorPlacement.EquallySpacedRectSide\",\"uuid\":\"8698242e-d004-4fda-889c-69f0784e7402\"},{\"content\":{\"connectorIds\":[],\"side\":\"TOP\"},\"type\":\"ConnectorPlacement.EquallySpacedRectSide\",\"uuid\":\"7829013b-7288-42bb-bccf-7e6edbe20d12\"},{\"content\":{\"connectorIds\":[\"In2\"],\"side\":\"BOTTOM\"},\"type\":\"ConnectorPlacement.EquallySpacedRectSide\",\"uuid\":\"357a4631-0a09-454f-b0f2-2b693ca62a9f\"},{\"content\":{\"connectorIds\":[],\"side\":\"HIDDEN\"},\"type\":\"ConnectorPlacement.EquallySpacedRectSide\",\"uuid\":\"b5eacf60-b578-4936-bef0-d59a279d5824\"}]},\"type\":\"ConnectorPlacement.EquallySpacedConnector\",\"uuid\":\"d2ebf12e-a3e7-4a55-b8c6-fa4e5ed13b89\"}],\"packageUris\":[\"http://schema.mathworks.com/mf0/Connector/R2020b\"],\"version\":\"1.0\"}"
  Trq Split Fac : Subsystem
  TrqCtrl : Outport
  wires:
  Bus Creator4/1 -> Brake/Motor Trq Split/2(TrqLimit)
  Charge/Discharge Limit/2(MaxChrgTrq) -> Bus Creator4/2  "MaxChrgTrq"
  Trq Split Fac/1(DrvMd) -> Bus Creator3/2
  Trq Split Fac/2(TrqEM2fac) -> Bus Creator3/3
  Trq Split Fac/3(TrqEM1fac) -> Bus Creator3/4
  Brake/Motor Trq Split/2(BrkTrq) -> Mech. Brake Model/2(BrkTrq)
  [BreakOn] -> Mech. Brake Model/1(BreakOn)
  [Volt] -> Charge/Discharge Limit/3(BatVolt)
  [BatTemp] -> Charge/Discharge Limit/4(BatTemp)
  Brake/Motor Trq Split/1(TorqueCmd) -> Bus Creator3/1, [TrqCmd]  "TorqueCmd"
  [BatSoC] -> Charge/Discharge Limit/5(BatSoC)
  [MotorSpd] -> Charge/Discharge Limit/2(MotorSpd)
  Mech. Brake Model/1(BrakeForce) -> Bus Creator1/1  "BrakeForce"
  TrqReq/1 -> Brake/Motor Trq Split/1(TrqReq), Charge/Discharge Limit/1(TrqReq)
  [TrqCmd] -> Trq Split Fac/1(Tq)
  Charge/Discharge Limit/1(MaxDchTorque) -> Bus Creator4/1  "MaxDchTorque"
  Bus Creator3/1 -> Bus Creator1/2  "MotorCtrl"
  Charge/Discharge Limit/3(BreakOn) -> Brake/Motor Trq Split/3(BreakOn), [BreakOn]
  Bus Creator1/1 -> TrqCtrl/1
  Bus Selector/3 -> [BatTemp]  "<CellTemp>"
  Bus Selector/2 -> [Volt]  "<BatVolt>"
  Bus Selector/4 -> [BatSoC]  "<maxSoC>"
  Bus Selector/1 -> [MotorSpd]  "<EM1rpm>"
  Crtl/1 -> Bus Selector/1

== system BEVplantModel/Controller/Vehicle Control/Torque Req ==
  TrqCtrl : Inport
  Bus Creator : BusCreator  Inputs=2
  Bus Selector1 : BusSelector  OutputSignals=BrakeForce,MotorCtrl.TrqEM2fac,MotorCtrl.TorqueCmd,MotorCtrl.TrqEM1fac
  Product1 : Product
  Product2 : Product
  TrqCmd : Outport
  BrakeCmd : Outport  Port=2
  wires:
  Bus Selector1/3 -> Product1/1, Product2/2  "<TorqueCmd>"
  Product1/1 -> Bus Creator/2  "EM1Trq"
  Product2/1 -> Bus Creator/1  "EM2Trq"
  TrqCtrl/1 -> Bus Selector1/1
  Bus Selector1/2 -> Product2/1  "<TrqEM2fac>"
  Bus Selector1/4 -> Product1/2  "<TrqEM1fac>"
  Bus Creator/1 -> TrqCmd/1
  Bus Selector1/1 -> BrakeCmd/1  "<BrakeForce>"

== system BEVplantModel/Vehicle/Battery Pump/Pump Demand ==
  No current : fl_lib/Physical Signals/Sources/PS Constant  constant=0 A
  PS Abs : fl_lib/Physical Signals/Nonlinear Operators/PS Abs
      settings: InternalSimscapePortConfiguration="{\"Bottom\":[],\"Left\":[{\"id\":\"I\",\"label\":\"\",\"type\":\"input\"}],\"Right\":[{\"id\":\"O\",\"label\":\"\",\"type\":\"output\"}],\"Top\":[]}"
  PS Divide : fl_lib/Physical Signals/Functions/PS Divide
  PS Product : fl_lib/Physical Signals/Functions/PS Product
  PS Switch : fl_lib/Physical Signals/Nonlinear Operators/PS Switch  Threshold=0.5
      settings: InternalSimscapePortConfiguration="{\"Bottom\":[],\"Left\":[{\"id\":\"I1\",\"label\":\"\",\"type\":\"input\"},{\"id\":\"I2\",\"label\":\"\",\"type\":\"input\"},{\"id\":\"I3\",\"label\":\"\",\"type\":\"input\"}],\"Right\":[{\"id\":\"O\",\"label\":\"\",\"type\":\"output\"}],\"Top\":[]}"
  PS Switch1 : fl_lib/Physical Signals/Nonlinear Operators/PS Switch  Threshold=0.5
      settings: InternalSimscapePortConfiguration="{\"Bottom\":[],\"Left\":[{\"id\":\"I1\",\"label\":\"\",\"type\":\"input\"},{\"id\":\"I2\",\"label\":\"\",\"type\":\"input\"},{\"id\":\"I3\",\"label\":\"\",\"type\":\"input\"}],\"Right\":[{\"id\":\"O\",\"label\":\"\",\"type\":\"output\"}],\"Top\":[]}"
  Zero Divide Protection : fl_lib/Physical Signals/Sources/PS Constant  constant=1 V
  BatSt : PMIOPort  Side=Left
  Volt : PMIOPort  Port=2  Side=Left
  Q : PMIOPort  Port=3  Side=Left
  P : PMIOPort  Port=4  Side=Left
  I : PMIOPort  Port=5  Side=Right
  connections:
  No current/RConn1 -- PS Switch/LConn3
  PS Switch1/LConn1 -- Volt/RConn1
  PS Switch/LConn1 -- PS Divide/RConn1
  BatSt/RConn1 -- PS Switch/LConn2 -- PS Switch1/LConn2
  PS Switch/RConn1 -- I/RConn1
  PS Divide/LConn1 -- PS Product/RConn1
  PS Abs/RConn1 -- PS Product/LConn2
  Q/RConn1 -- PS Product/LConn1
  P/RConn1 -- PS Abs/LConn1
  PS Switch1/RConn1 -- PS Divide/LConn2
  Zero Divide Protection/RConn1 -- PS Switch1/LConn3

== system BEVplantModel/Vehicle/Battery Pump/current sensing1 ==
  Current Sensor : fl_lib/Electrical/Electrical Sensors/Current Sensor
  PS-Simulink Converter : nesl_utility/PS-Simulink Converter  PhysicalDomain=network_engine_domain  SubClassName=ps_output  LeftPortType=input  RightPortType=output  PseudoPeriodic=off  Frequencies=[]  VectorFormat=inherit  Unit=inherit  AffineConversion=off
  "  " : PMIOPort  Side=Left
  " " : PMIOPort  Port=2  Side=Right
  "   " : Outport
  wires:
  PS-Simulink Converter/1 -> "   "/1
  connections:
  PS-Simulink Converter/LConn1 -- Current Sensor/RConn1
  Current Sensor/LConn1 -- "  "/RConn1
  Current Sensor/RConn2 -- " "/RConn1

== system BEVplantModel/Vehicle/Chiller/Chiller Subsystem ==
  BattSt : Inport
  ThCtrl : Inport  Port=2
  Chiller Demand : Subsystem
  Compare To Constant : simulink/Logic and Bit Operations/Compare To Constant  relop=>  const=0  OutDataTypeStr=boolean
  Constant1 : Constant  Value=0
  Constant2 : Constant
  Max Power [W] : Gain  Gain=-vehicleThermal.chillerMaxPower
  Product : Product
  Simulink-PS Converter : nesl_utility/Simulink-PS Converter  PhysicalDomain=network_engine_domain  SubClassName=ps_input  LeftPortType=input  RightPortType=output  PseudoPeriodic=off  Frequencies=[]  NoiseDistribution=none  NoiseParameters=[]  Unit=W  AffineConversion=off  FilteringAndDerivatives=provide  SimscapeFilterOrder=1  InputFilterTimeConstant=0.001  UdotUserProvided=0
  Simulink-PS Converter2 : nesl_utility/Simulink-PS Converter  PhysicalDomain=network_engine_domain  SubClassName=ps_input  LeftPortType=input  RightPortType=output  PseudoPeriodic=off  Frequencies=[]  NoiseDistribution=none  NoiseParameters=[]  Unit=1  AffineConversion=off  FilteringAndDerivatives=provide  SimscapeFilterOrder=1  InputFilterTimeConstant=0.001  UdotUserProvided=0
  Switch : Switch  Criteria=u2 > Threshold  SaturateOnIntegerOverflow=off  InputSameDT=off
  Transfer Fcn : TransferFcn  Denominator=[1 1]
  V : PMIOPort  Side=Left
  I : PMIOPort  Port=2  Side=Right
  output : PMIOPort  Port=3  Side=Right
  wires:
  Max Power [W]/1 -> Product/2
  Switch/1 -> Transfer Fcn/1
  ThCtrl/1 -> Switch/2
  Transfer Fcn/1 -> Max Power [W]/1
  BattSt/1 -> Compare To Constant/1, Simulink-PS Converter2/1
  Product/1 -> Simulink-PS Converter/1
  Compare To Constant/1 -> Product/1
  Constant2/1 -> Switch/3
  Constant1/1 -> Switch/1
  connections:
  Simulink-PS Converter/RConn1 -- output/RConn1 -- Chiller Demand/LConn3
  Chiller Demand/LConn1 -- V/RConn1
  Chiller Demand/LConn2 -- Simulink-PS Converter2/RConn1
  Chiller Demand/RConn1 -- I/RConn1

== system BEVplantModel/Vehicle/Chiller/current sensing1 ==
  Current Sensor : fl_lib/Electrical/Electrical Sensors/Current Sensor
  PS-Simulink Converter : nesl_utility/PS-Simulink Converter  PhysicalDomain=network_engine_domain  SubClassName=ps_output  LeftPortType=input  RightPortType=output  PseudoPeriodic=off  Frequencies=[]  VectorFormat=inherit  Unit=inherit  AffineConversion=off
  "  " : PMIOPort  Side=Left
  " " : PMIOPort  Port=2  Side=Right
  "   " : Outport
  wires:
  PS-Simulink Converter/1 -> "   "/1
  connections:
  PS-Simulink Converter/LConn1 -- Current Sensor/RConn1
  Current Sensor/LConn1 -- "  "/RConn1
  Current Sensor/RConn2 -- " "/RConn1

== system BEVplantModel/Vehicle/Chiller Bypass Valve/Valve Control ==
  ThCtrl : Inport
  Bias : Bias  Bias=-1  SaturateOnIntegerOverflow=off
  Gain : Gain  Gain=2
  Max Valve Displacement [m] : Gain  Gain=vehicleThermal.coolant_valve_displacement
  Simulink-PS Converter : nesl_utility/Simulink-PS Converter  PhysicalDomain=network_engine_domain  SubClassName=ps_input  LeftPortType=input  RightPortType=output  PseudoPeriodic=off  Frequencies=[]  NoiseDistribution=none  NoiseParameters=[]  Unit=m  AffineConversion=off  FilteringAndDerivatives=provide  SimscapeFilterOrder=1  InputFilterTimeConstant=0.001  UdotUserProvided=0
  Transfer Fcn : TransferFcn  Denominator=[1 1]
  Disp : PMIOPort  Side=Right
  wires:
  Gain/1 -> Bias/1
  Bias/1 -> Max Valve Displacement [m]/1
  Max Valve Displacement [m]/1 -> Simulink-PS Converter/1
  ThCtrl/1 -> Transfer Fcn/1
  Transfer Fcn/1 -> Gain/1
  connections:
  Simulink-PS Converter/RConn1 -- Disp/RConn1

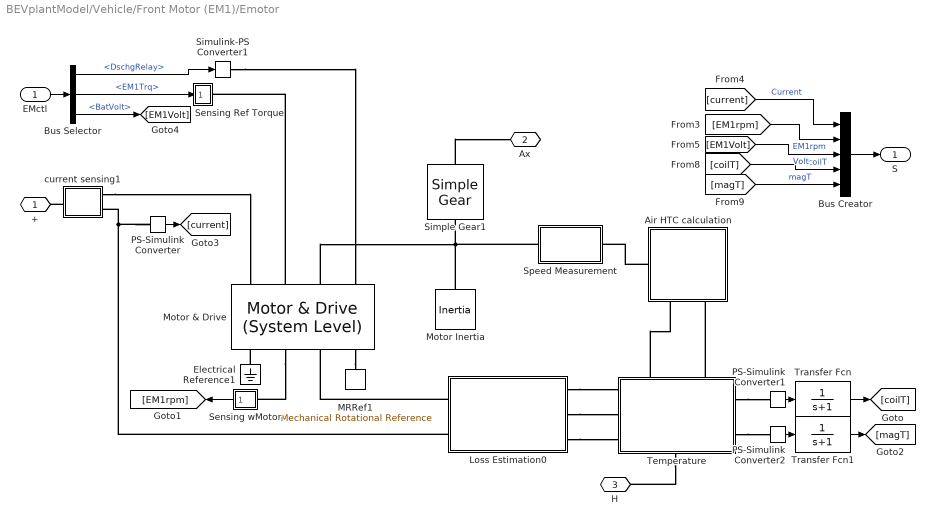
== system BEVplantModel/Vehicle/Front Motor (EM1)/Emotor ==
  EMctl : Inport
  Air HTC calculation : Subsystem
      settings: PortSchema="{\"entries\":[{\"content\":{\"sides\":[{\"content\":{\"connectorIds\":[\"LConn1\"]},\"type\":\"ConnectorPlacement.EquallySpacedRectSide\",\"uuid\":\"c3fc49c2-0151-484f-b0d8-f4e4a060bcaf\"},{\"content\":{\"connectorIds\":[],\"side\":\"RIGHT\"},\"type\":\"ConnectorPlacement.EquallySpacedRectSide\",\"uuid\":\"c73251fe-fcad-4c5f-9d27-fb7ac98c9b31\"},{\"content\":{\"connectorIds\":[],\"side\":\"TOP\"},\"type\":\"ConnectorPlacement.EquallySpacedRectSide\",\"uuid\":\"06ea8515-c1b4-4445-9ea2-9a6fe3b8d822\"},{\"content\":{\"connectorIds\":[\"RConn1\",\"RConn2\"],\"side\":\"BOTTOM\"},\"type\":\"ConnectorPlacement.EquallySpacedRectSide\",\"uuid\":\"0d77474d-64a7-49ab-b2b5-eb3962b26dfa\"}]},\"type\":\"ConnectorPlacement.EquallySpacedConnector\",\"uuid\":\"651eda7a-2416-4496-9b8b-1b2d725cf6dd\"}],\"packageUris\":[\"http://schema.mathworks.com/mf0/Connector/R2020b\"],\"version\":\"1.0\"}"
  Bus Creator : BusCreator  Inputs=5
  Bus Selector : BusSelector  OutputSignals=DschgRelay,EM1Trq,BattSensor.BatVolt
  Electrical Reference1 : fl_lib/Electrical/Electrical Elements/Electrical Reference
  Loss Estimation0 : Subsystem
  MRRef1 : fl_lib/Mechanical/Rotational Elements/Mechanical Rotational Reference
  Motor & Drive : ee_lib/Electromechanical/Motor & Drive (System Level)  torque_speed_param=2  overtorque_param=ee.enum.electromech.overtorque.no  T_t=[max_torque max_torque max_torque 0] N*m  T_t_intermittent=[.36, .32, .28, 0] N*m  T_t_2D=[.09, .09, .09; .08, .08, .08; .07, .07, .07; 0, 0, 0] N*m  T_t_intermittent_2D=[.36, .36, .36; .32, .32, .32; .28, .28, .28; 0, 0, 0] N*m  w_t=[ 0 3.75e+3 7.5e+3 8e+3 ] rpm  vdc_t=[6, 12, 24] V  torque_max=electricDrive.max_torque N*m  power_max=electricDrive.max_power W  torque_max_intermittent=0.4 N*m  power_max_intermittent=120 W  time_overtorque=30 s  time_recover=60 s  Tc=electricDrive.Tctc s  losses_param=2  eff=96  w_eff=1500 rpm  T_eff=50 N*m  Piron=200 W  Pbase=0 W  w_eff_vec=electricDrive.loss_maps.spMat rpm  T_eff_vec=electricDrive.loss_maps.tqMat N*m  v_eff_vec=[100, 250, 400] V  losses_mat=electricDrive.loss_maps.lossMat W  efficiency_mat=[95 95 95 95; 95 95 95 95; 95 95 95 95; 95 95 95 95; 95 95 95 95]  losses_mat_3D=ones(5, 4, 3) W  efficiency_mat_3D=95 * ones(5, 4, 3)  Res=0 Ohm  enable_fault=simscape.enum.onoff.on  fault_condition=1  fault_threshold=0.5  J=0 kg*m^2  lam=1e-5 N*m/(rad/s)  speed0=0 rpm  faulted_specify=off  faulted_priority=None  faulted=0  faulted_nominal_specify=off  faulted_nominal_unit=1  faulted_nominal_value=1  torqueLimitContinuous_specify=off  torqueLimitContinuous_priority=None  torqueLimitContinuous=0 N*m  torqueLimitContinuous_nominal_specify=off  torqueLimitContinuous_nominal_unit=N*m  torqueLimitContinuous_nominal_value=1  alpha=0.00393 1/K  Tmeas=30 degC  Tmeas2=31 degC  losses_mat_T2=electricDrive.loss_maps.lossMat W  efficiency_mat_T2=[95 95 95 95; 95 95 95 95; 95 95 95 95; 95 95 95 95; 95 95 95 95]  losses_mat_3D_T2=ones(5, 4, 3) W  efficiency_mat_3D_T2=95 * ones(5, 4, 3)  thermal_mass=15000 J/K  initial_temperature=vehicleThermal.coolant_T_init K
      settings: InternalSimscapePortConfiguration="{\"Bottom\":[],\"Left\":[{\"id\":\"Vp\",\"label\":\"+\",\"type\":\"foundation.electrical.electrical\"},{\"id\":\"Tr\",\"label\":\"Tr\",\"type\":\"input\"},{\"id\":\"R\",\"label\":\"R\",\"type\":\"foundation.mechanical.rotational.rotational\"},{\"id\":\"F\",\"label\":\"F\",\"type\":\"input\"}],\"Right\":[{\"id\":\"Vm\",\"label\":\"-\",\"type\":\"foundation.electrical.electrical\"},{\"id\":\"Omega\",\"label\":\"w\",\"type\":\"output\"},{\"id\":\"H\",\"label\":\"H\",\"type\":\"foundation.thermal.thermal\"},{\"id\":\"C\",\"label\":\"C\",\"type\":\"foundation.mechanical.rotational.rotational\"}],\"Top\":[]}"
  Motor Inertia : fl_lib/Mechanical/Rotational Elements/Inertia  inertia=0.02 kg*m^2  num_ports=foundation.enum.numPorts2.one  w_specify=on  w_priority=High  w=0 rpm  w_nominal_specify=off  w_nominal_unit=rad/s  w_nominal_value=1  t_specify=off  t_priority=High  t=0 N*m  t_nominal_specify=off  t_nominal_unit=N*m  t_nominal_value=1
  PS-Simulink Converter : nesl_utility/PS-Simulink Converter  PhysicalDomain=network_engine_domain  SubClassName=ps_output  LeftPortType=input  RightPortType=output  PseudoPeriodic=off  Frequencies=[]  VectorFormat=inherit  Unit=inherit  AffineConversion=off
  PS-Simulink Converter1 : nesl_utility/PS-Simulink Converter  PhysicalDomain=network_engine_domain  SubClassName=ps_output  LeftPortType=input  RightPortType=output  PseudoPeriodic=off  Frequencies=[]  VectorFormat=inherit  Unit=inherit  AffineConversion=off
  PS-Simulink Converter2 : nesl_utility/PS-Simulink Converter  PhysicalDomain=network_engine_domain  SubClassName=ps_output  LeftPortType=input  RightPortType=output  PseudoPeriodic=off  Frequencies=[]  VectorFormat=inherit  Unit=inherit  AffineConversion=off
  Sensing Ref Torque : Subsystem
  Sensing wMotor : Subsystem
      mask Display: disp('rpm');
  Simple Gear1 : sdl_lib/Gears/Simple Gear  ratio=0.3  rotation_direction=sdl.enum.shaftOutputDirection.same  friction_model=sdl.enum.gear_efficiencies_load.off  T_noload=0.1 N*m  T_nom=5 N*m  efficiency_nom=0.8  efficiency=0.8  temperature_TLU=[280, 300, 320] K  load_TLU=[1, 5, 10] N*m  efficiency_TLU=[.95, .9, .85]  efficiency_TLU2=[.85, .8, .75; .95, .9, .85; .85, .8, .7]  w_thr=0.01 rad/s  pwr_thr=0.001 W  backlash_model=sdl.enum.backlashModel.Off  backlash_distance=1e-3 mm  x0=0 mm  r_base=0.1 m  hardstop_model=simscape.enum.hardstop.smooth  transition=1e-4 mm  backlash_stiffness=1e7 N/m  backlash_damping=1e6 N*s/m  e=0  v_tol=0.001 m/s  mu_visc=[0, 0] N*m*s/rad  enable_faults=simscape.enum.onoff.off  efficiency_fault=0.05  external_fault=simscape.enum.onoff.off  temporal_fault=simscape.enum.onoff.off  fault_time=5 s  fault_angles=pi / 12 rad  report_fault=simscape.enum.assert.action.none  thermal_mass=50 J/K  temperature_specify=off  temperature_priority=High  temperature=300 K  temperature_nominal_specify=off  temperature_nominal_unit=K  temperature_nominal_value=1  x_backlash_specify=off  x_backlash_priority=None  x_backlash=0 mm  x_backlash_nominal_specify=off  x_backlash_nominal_unit=mm  x_backlash_nominal_value=1  f_hardstop_specify=off  f_hardstop_priority=None  f_hardstop=0 N  f_hardstop_nominal_specify=off  f_hardstop_nominal_unit=N  f_hardstop_nominal_value=1  v_backlash_specify=off  v_backlash_priority=None  v_backlash=0 m/s  v_backlash_nominal_specify=off  v_backlash_nominal_unit=m/s  v_backlash_nominal_value=1
  Simulink-PS Converter1 : nesl_utility/Simulink-PS Converter  PhysicalDomain=network_engine_domain  SubClassName=ps_input  LeftPortType=input  RightPortType=output  PseudoPeriodic=off  Frequencies=[]  NoiseDistribution=none  NoiseParameters=[]  Unit=1  AffineConversion=off  FilteringAndDerivatives=provide  SimscapeFilterOrder=1  InputFilterTimeConstant=0.001  UdotUserProvided=0
  Speed Measurement : Subsystem
  Temperature : Subsystem
      settings: PortSchema="{\"entries\":[{\"content\":{\"sides\":[{\"content\":{\"connectorIds\":[\"LConn1\",\"LConn2\",\"LConn3\"]},\"type\":\"ConnectorPlacement.EquallySpacedRectSide\",\"uuid\":\"fee72484-960d-4cd4-9296-e38678962aa1\"},{\"content\":{\"connectorIds\":[\"RConn1\",\"RConn2\"],\"side\":\"RIGHT\"},\"type\":\"ConnectorPlacement.EquallySpacedRectSide\",\"uuid\":\"5fc115b4-63fd-47d3-871d-1c82ac52ac43\"},{\"content\":{\"connectorIds\":[\"LConn4\",\"LConn5\"],\"side\":\"TOP\"},\"type\":\"ConnectorPlacement.EquallySpacedRectSide\",\"uuid\":\"406f719a-f995-4122-9f35-24e8332a2e84\"},{\"content\":{\"connectorIds\":[\"RConn3\"],\"side\":\"BOTTOM\"},\"type\":\"ConnectorPlacement.EquallySpacedRectSide\",\"uuid\":\"14dc85e6-8157-4b38-8651-862ce77721cd\"}]},\"type\":\"ConnectorPlacement.EquallySpacedConnector\",\"uuid\":\"1dcc2b5d-90fd-40de-873d-99118eb86bdd\"}],\"packageUris\":[\"http://schema.mathworks.com/mf0/Connector/R2020b\"],\"version\":\"1.0\"}"
  Transfer Fcn : TransferFcn  Denominator=[1 1]
  Transfer Fcn1 : TransferFcn  Denominator=[1 1]
  current sensing1 : Subsystem
  + : PMIOPort  Side=Left
  "Ax  " : PMIOPort  Port=2  Side=Right
  H : PMIOPort  Port=3  Side=Right
  S : Outport
  wires:
  Sensing wMotor/1(SL) -> [EM1rpm]
  PS-Simulink Converter/1 -> [current]
  [magT] -> Bus Creator/5  "magT"
  [current] -> Bus Creator/1  "Current"
  Bus Creator/1 -> S/1
  [EM1rpm] -> Bus Creator/2  "EM1rpm"
  [coilT] -> Bus Creator/4  "coilT"
  [EM1Volt] -> Bus Creator/3  "Volt"
  Bus Selector/1 -> Simulink-PS Converter1/1  "<DschgRelay>"
  Bus Selector/3 -> [EM1Volt]  "<BatVolt>"
  EMctl/1 -> Bus Selector/1
  Bus Selector/2 -> Sensing Ref Torque/1(" ")  "<EM1Trq>"
  Transfer Fcn1/1 -> [magT]
  Transfer Fcn/1 -> [coilT]
  PS-Simulink Converter1/1 -> Transfer Fcn/1
  PS-Simulink Converter2/1 -> Transfer Fcn1/1
  connections:
  Motor & Drive/RConn4 -- MRRef1/LConn1
  current sensing1/RConn1 -- Motor & Drive/LConn1
  Motor Inertia/LConn1 -- Speed Measurement/LConn1 -- Simple Gear1/RConn1 -- Motor & Drive/LConn3
  Simple Gear1/LConn1 -- "Ax  "/RConn1
  current sensing1/LConn1 -- +/RConn1
  Temperature/RConn3 -- H/RConn1
  Loss Estimation0/RConn2 -- Temperature/LConn2
  Motor & Drive/LConn2 -- Sensing Ref Torque/RConn1
  Motor & Drive/RConn2 -- Sensing wMotor/LConn1
  Air HTC calculation/LConn1 -- Speed Measurement/RConn1
  Loss Estimation0/RConn3 -- Temperature/LConn3
  Electrical Reference1/LConn1 -- Motor & Drive/RConn1
  Simulink-PS Converter1/RConn1 -- Motor & Drive/LConn4
  Loss Estimation0/LConn1 -- Motor & Drive/RConn3
  Loss Estimation0/RConn1 -- Temperature/LConn1
  Temperature/LConn4 -- Air HTC calculation/RConn1
  Temperature/LConn5 -- Air HTC calculation/RConn2
  Temperature/RConn1 -- PS-Simulink Converter1/LConn1
  Temperature/RConn2 -- PS-Simulink Converter2/LConn1
  PS-Simulink Converter/LConn1 -- Loss Estimation0/LConn2 -- current sensing1/RConn2

== system BEVplantModel/Vehicle/Front Motor (EM1)/Emotor Input ==
  "Tq  " : Inport
  "Batt " : Inport  Port=2
  Bus Creator : BusCreator  Inputs=3
  Bus Selector3 : BusSelector  OutputSignals=Relay.RelayDchg,BattSensor
  Constant : Constant
  Constant1 : Constant  Value=0
  Switch : Switch  Criteria=u2 > Threshold  SaturateOnIntegerOverflow=off  InputSameDT=off
  EMctl : Outport
  wires:
  "Tq  "/1 -> Bus Creator/1
  Switch/1 -> Bus Creator/2  "DschgRelay"
  Constant1/1 -> Switch/1
  Constant/1 -> Switch/3
  Bus Selector3/1 -> Switch/2  "<RelayDchg>"
  "Batt "/1 -> Bus Selector3/1
  Bus Creator/1 -> EMctl/1
  Bus Selector3/2 -> Bus Creator/3  "<BattSensor>"

== system BEVplantModel/Vehicle/Front Motor (EM1)/Emotor Output ==
  S : Inport
  Bus Selector1 : BusSelector  OutputSignals=Current,Volt
  Constant : Constant  Value=3600
  Divide : Product  Inputs=*/
  Integrator : Integrator
  Product : Product
  EM1 : Outport
  E : Outport  Port=2
  wires:
  Divide/1 -> E/1  "EM1energy"
  Constant/1 -> Divide/2
  Integrator/1 -> Divide/1
  Product/1 -> Integrator/1
  S/1 -> EM1/1, Bus Selector1/1  "EM1sensor"
  Bus Selector1/2 -> Product/2  "<Volt>"
  Bus Selector1/1 -> Product/1  "<Current>"
